simulink model "posctrl"  (R2013a)
settings: Solver=ode23tb  StartTime=0.0  StopTime=1.6*T  RelTol=1e-4
values from neighbouring files (symbols this model uses):
  Cf = 1e-3    (= 0.001)    [dimensionamento.m]
  ftr = 10e3    (= 10000)    [dimensionamento.m]
  g = 10    [dimensionamento.m]
  Irob = m*l^2/3    (= 0.48)    [dimensionamento.m]
  J = 2.22e-2    (= 0.0222)    [dimensionamento.m]
  kt = kt1    [dimensionamento.m]
  l = 0.60    (= 0.6)    [dimensionamento.m]
  La = 28e-3    (= 0.028)    [dimensionamento.m]
  m = 4    [dimensionamento.m]
  Ra = 2.58    [dimensionamento.m]
  reduc = 1    [dimensionamento.m]
  T = 10    [dimensionamento.m]
  thetaf = 90    [dimensionamento.m]
  thetai = 0    [dimensionamento.m]
  Tnom = Pnom/Wnom    (= 20.3454584681)    [dimensionamento.m]
  Vsource = Vnom    (= 240)    [dimensionamento.m]
libraries: powerlib x9, simulink x6
settings Model: Creator=dello  LastModifiedBy=dello
settings SolverCC: SolverResetMethod=Robust
settings DataIOCC: SignalLoggingSaveFormat=ModelDataLogs  SignalLoggingName=results

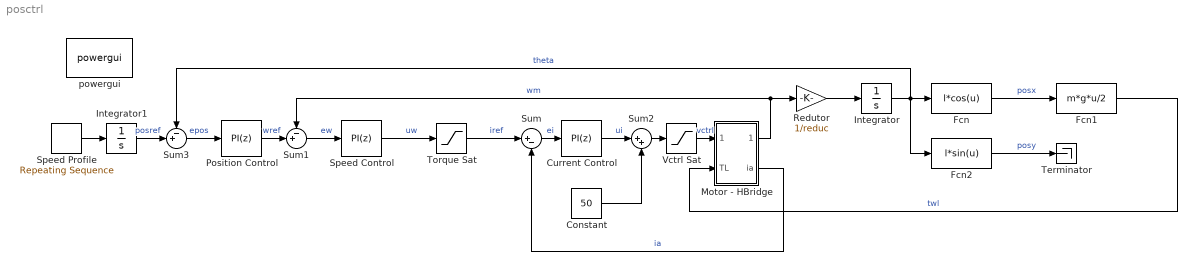
== system posctrl ==
  Constant : Constant  Value=50
  Current Control : simulink/Continuous/PID Controller  Controller=PI  TimeDomain=Discrete-time  SampleTime=1e-3  IntegratorMethod=Forward Euler  FilterMethod=Forward Euler  Form=Parallel  P=3  I=100  D=0  N=100  InitialConditionSource=internal  InitialConditionForIntegrator=0  InitialConditionForFilter=0  ExternalReset=none  LimitOutput=off  UpperSaturationLimit=inf  LowerSaturationLimit=-inf  LinearizeAsGain=on  AntiWindupMode=none  Kb=1  TrackingMode=off  Kt=1  PParamMin=[]  PParamMax=[]  IParamMin=[]  IParamMax=[]  DParamMin=[]  DParamMax=[]  NParamMin=[]  NParamMax=[]  KbParamMin=[]  KbParamMax=[]  KtParamMin=[]  KtParamMax=[]  POutMin=[]  POutMax=[]  IOutMin=[]  IOutMax=[]  DOutMin=[]  DOutMax=[]  NOutMin=[]  NOutMax=[]  KbOutMin=[]  KbOutMax=[]  KtOutMin=[]  KtOutMax=[]  IntegratorOutMin=[]  IntegratorOutMax=[]  FilterOutMin=[]  FilterOutMax=[]  SumOutMin=[]  SumOutMax=[]  SumI1OutMin=[]  SumI1OutMax=[]  SumI2OutMin=[]  SumI2OutMax=[]  SumI3OutMin=[]  SumI3OutMax=[]  SumDOutMin=[]  SumDOutMax=[]  SaturationOutMin=[]  SaturationOutMax=[]  IntegratorContinuousStateAttributes=''  IntegratorStateMustResolveToSignalObject=off  IntegratorRTWStateStorageClass=Auto  FilterContinuousStateAttributes=''  FilterStateMustResolveToSignalObject=off  FilterRTWStateStorageClass=Auto
  Fcn : Fcn  Expr=l*cos(u)
  Fcn1 : Fcn  Expr=m*g*u/2
  Fcn2 : Fcn  Expr=l*sin(u)
  Integrator : Integrator  InitialCondition=thetai  LimitOutput=on  UpperSaturationLimit=90  LowerSaturationLimit=0
  Integrator1 : Integrator  InitialCondition=thetai  UpperSaturationLimit=90  LowerSaturationLimit=0
  Motor - HBridge : Subsystem
  Position Control : simulink/Continuous/PID Controller  Controller=PI  TimeDomain=Discrete-time  SampleTime=1e-3  IntegratorMethod=Forward Euler  FilterMethod=Forward Euler  Form=Parallel  P=200  I=0  D=0  N=100  InitialConditionSource=internal  InitialConditionForIntegrator=0  InitialConditionForFilter=0  ExternalReset=none  LimitOutput=off  UpperSaturationLimit=inf  LowerSaturationLimit=-inf  LinearizeAsGain=on  AntiWindupMode=none  Kb=1  TrackingMode=off  Kt=1  PParamMin=[]  PParamMax=[]  IParamMin=[]  IParamMax=[]  DParamMin=[]  DParamMax=[]  NParamMin=[]  NParamMax=[]  KbParamMin=[]  KbParamMax=[]  KtParamMin=[]  KtParamMax=[]  POutMin=[]  POutMax=[]  IOutMin=[]  IOutMax=[]  DOutMin=[]  DOutMax=[]  NOutMin=[]  NOutMax=[]  KbOutMin=[]  KbOutMax=[]  KtOutMin=[]  KtOutMax=[]  IntegratorOutMin=[]  IntegratorOutMax=[]  FilterOutMin=[]  FilterOutMax=[]  SumOutMin=[]  SumOutMax=[]  SumI1OutMin=[]  SumI1OutMax=[]  SumI2OutMin=[]  SumI2OutMax=[]  SumI3OutMin=[]  SumI3OutMax=[]  SumDOutMin=[]  SumDOutMax=[]  SaturationOutMin=[]  SaturationOutMax=[]  IntegratorContinuousStateAttributes=''  IntegratorStateMustResolveToSignalObject=off  IntegratorRTWStateStorageClass=Auto  FilterContinuousStateAttributes=''  FilterStateMustResolveToSignalObject=off  FilterRTWStateStorageClass=Auto
  Redutor : Gain  Gain=1/reduc
  Speed Control : simulink/Continuous/PID Controller  Controller=PI  TimeDomain=Discrete-time  SampleTime=1e-3  IntegratorMethod=Forward Euler  FilterMethod=Forward Euler  Form=Parallel  P=10  I=1  D=0  N=100  InitialConditionSource=internal  InitialConditionForIntegrator=0  InitialConditionForFilter=0  ExternalReset=none  LimitOutput=off  UpperSaturationLimit=inf  LowerSaturationLimit=-inf  LinearizeAsGain=on  AntiWindupMode=none  Kb=1  TrackingMode=off  Kt=1  PParamMin=[]  PParamMax=[]  IParamMin=[]  IParamMax=[]  DParamMin=[]  DParamMax=[]  NParamMin=[]  NParamMax=[]  KbParamMin=[]  KbParamMax=[]  KtParamMin=[]  KtParamMax=[]  POutMin=[]  POutMax=[]  IOutMin=[]  IOutMax=[]  DOutMin=[]  DOutMax=[]  NOutMin=[]  NOutMax=[]  KbOutMin=[]  KbOutMax=[]  KtOutMin=[]  KtOutMax=[]  IntegratorOutMin=[]  IntegratorOutMax=[]  FilterOutMin=[]  FilterOutMax=[]  SumOutMin=[]  SumOutMax=[]  SumI1OutMin=[]  SumI1OutMax=[]  SumI2OutMin=[]  SumI2OutMax=[]  SumI3OutMin=[]  SumI3OutMax=[]  SumDOutMin=[]  SumDOutMax=[]  SaturationOutMin=[]  SaturationOutMax=[]  IntegratorContinuousStateAttributes=''  IntegratorStateMustResolveToSignalObject=off  IntegratorRTWStateStorageClass=Auto  FilterContinuousStateAttributes=''  FilterStateMustResolveToSignalObject=off  FilterRTWStateStorageClass=Auto
  Speed Profile : simulink/Sources/Repeating Sequence  rep_seq_t="[0 0.3*T 0.4*T 1.2*T  1.3*T 1.6*T]"  rep_seq_y=[0 0 (thetaf - thetai)/180*pi/0.9/T (thetaf - thetai)/180*pi/0.9/T 0 0]
  Sum : Sum  Inputs=|+-
  Sum1 : Sum  Inputs=-+|
  Sum2 : Sum  Inputs=|++
  Sum3 : Sum  Inputs=-+|
  Terminator : Terminator
  Torque Sat : Saturate  UpperLimit=Tnom/kt  LowerLimit=-Tnom/kt
  Vctrl Sat : Saturate  UpperLimit=100  LowerLimit=0
  powergui : powerlib/powergui  Priority=1  SimulationMode=Continuous  SolverType=Tustin  SampleTime=50e-6  frequency=60  SPID=off  DisableSnubberDevices=off  DisableRonSwitches=off  DisableVfSwitches=off  SwTol=0  Interpol=off  DisplayEquations=off  frequencyindice=0  Pbase=100e6  ErrMax=1e-4  Iterations=50  UnitsV=kV  UnitsW=MW  FunctionMessages=off  echomessages=off  HookPort=off  EnableUseOfTLC=off  x0status=blocks  RestoreLinks=warning  ResistiveCurrentMeasurement=off  Frange=[0:2:500]  Ylog=off  Xlog=on  ShowGrid=off  save=off  variable=ZData  ZoomFFT=off  StartTime=0.0  cycles=1  DisplayStyle=1  fundamental=60  FreqAxis=off  MaxFrequency=1000  frequencyindicesteady=1  RmsSteady=1  display=off  Ts=0  methode=off
  wires:
  Vctrl Sat/1 -> Motor - HBridge/1(vctrl)  "vctrl"
  Motor - HBridge/2(ia) -> Sum/2  "ia"
  Sum/1 -> Current Control/1  "ei"
  Current Control/1 -> Sum2/1  "ui"
  Motor - HBridge/1(wm) -> Redutor/1, Sum1/1  "wm"
  Sum1/1 -> Speed Control/1  "ew"
  Speed Control/1 -> Torque Sat/1  "uw"
  Torque Sat/1 -> Sum/1  "iref"
  Constant/1 -> Sum2/2
  Sum2/1 -> Vctrl Sat/1
  Integrator/1 -> Sum3/1, Fcn2/1, Fcn/1  "theta"
  Fcn/1 -> Fcn1/1  "posx"
  Fcn1/1 -> Motor - HBridge/2(TL)  "twl"
  Fcn2/1 -> Terminator/1  "posy"
  Speed Profile/1 -> Integrator1/1
  Sum3/1 -> Position Control/1  "epos"
  Position Control/1 -> Sum1/2  "wref"
  Integrator1/1 -> Sum3/2  "posref"
  Redutor/1 -> Integrator/1

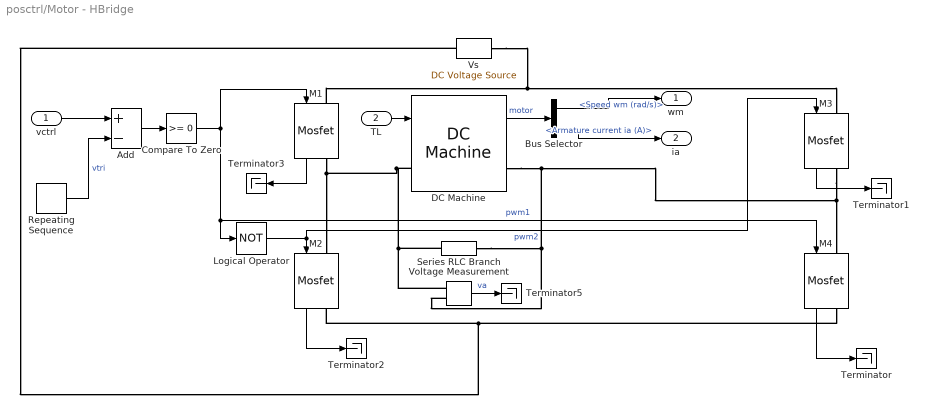
== system posctrl/Motor - HBridge ==
  vctrl : Inport
  TL : Inport  Port=2
  Add : Sum  Inputs=+-
  Bus Selector : BusSelector  OutputSignals=Speed wm (rad/s),Armature current ia (A)
  Compare To Zero : simulink/Logic and Bit Operations/Compare To Zero  relop=>=  OutDataTypeStr=boolean
  DC Machine : powerlib/Machines/DC Machine  PresetModel=No  MechanicalLoad=Torque TL  FieldType=Permanent magnet  ShowDetailedParameters=on  RLa=[ Ra La]  RLf="[ 240  120]"  Laf=1.8  MachineConstant=Torque constant (N.m/A)  Ke=1.8  Kt=kt  J=J + Irob/reduc  Bm=B  Tf=0  w0=0  Ifinit=1  TsPowergui=0  TsBlock=-1
  Logical Operator : Logic  Operator=NOT  IconShape=distinctive  AllPortsSameDT=off  OutDataTypeStr=boolean
  M{1..4} (4 alike) : powerlib/Power Electronics/Mosfet  Ron=0.1  Lon=0  Rd=0.01  Vfd=0  IC=0  Rs=1e5  Cs=inf  Measurements=on
  Repeating Sequence : simulink/Sources/Repeating Sequence  rep_seq_t=[0 1/ftr/2 1/ftr]  rep_seq_y=[0 100 0]
  Series RLC Branch : powerlib/Elements/Series RLC Branch  LConnTagsString=__new0  RConnTagsString=__new0  BranchType=C  Resistance=1  Inductance=1e-3  SetiL0=off  InitialCurrent=0  Capacitance=Cf  Setx0=off  InitialVoltage=0  Measurements=None
  Terminator{,1..3,5} (5 alike) : Terminator
  Voltage Measurement : powerlib/Measurements/Voltage Measurement  PhasorSimulation=off  OutputType=Complex  PSBequivalent=0
  Vs : powerlib/Electrical Sources/DC Voltage Source  Amplitude=Vsource  Measurements=None
  wm : Outport
  ia : Outport  Port=2
  wires:
  M1/1 -> Terminator3/1
  M3/1 -> Terminator1/1
  Repeating Sequence/1 -> Add/2  "vtri"
  vctrl/1 -> Add/1
  Add/1 -> Compare To Zero/1
  DC Machine/1 -> Bus Selector/1  "motor"
  Logical Operator/1 -> M2/1, M3/1  "pwm2"
  M2/1 -> Terminator2/1
  M4/1 -> Terminator/1
  Compare To Zero/1 -> M1/1, M4/1, Logical Operator/1  "pwm1"
  TL/1 -> DC Machine/1
  Voltage Measurement/1 -> Terminator5/1  "va"
  Bus Selector/2 -> ia/1  "<Armature current ia (A)>"
  Bus Selector/1 -> wm/1  "<Speed wm (rad/s)>"
  connections:
  M3/RConn1 -- Series RLC Branch/RConn1 -- Voltage Measurement/LConn2 -- DC Machine/RConn1 -- M4/LConn1
  M1/RConn1 -- Series RLC Branch/LConn1 -- Voltage Measurement/LConn1 -- DC Machine/LConn1 -- M2/LConn1
  M4/RConn1 -- Vs/LConn1 -- M2/RConn1
  M1/LConn1 -- Vs/RConn1 -- M3/LConn1
